simulink model "springScale_sith_weights"  (R2023a)
settings: Solver=VariableStepAuto  StartTime=0.0  StopTime=20.0  RelTol=1e-3
undefined symbols (not defined in the file or in its folder): c, k1, k2, m, x0
settings Model: Creator=kawat  LastModifiedBy=kawat

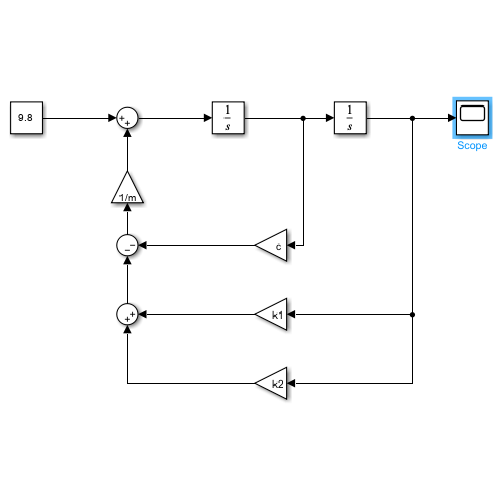
[thumbnail: Simulink's stored preview of the top-level diagram]
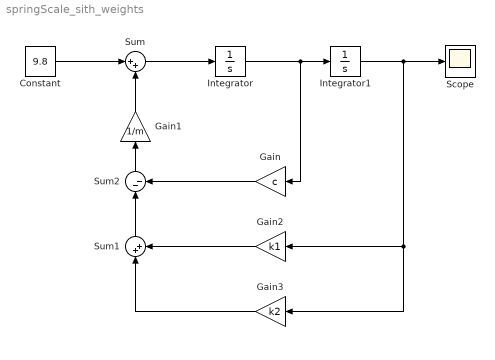
== system springScale_sith_weights ==
  Constant : Constant  Value=9.8  SampleTime=0.001
  Gain : Gain  Gain=c
  Gain1 : Gain  Gain=1/m
  Gain2 : Gain  Gain=k1
  Gain3 : Gain  Gain=k2
  Integrator : Integrator
  Integrator1 : Integrator  InitialCondition=x0
  Scope : Scope
  Sum : Sum  Inputs=|++
  Sum1 : Sum  Inputs=|++
  Sum2 : Sum  Inputs=|--
  wires:
  Constant/1 -> Sum/1
  Gain1/1 -> Sum/2
  Sum2/1 -> Gain1/1
  Sum1/1 -> Sum2/1
  Sum/1 -> Integrator/1
  Integrator/1 -> Gain/1, Integrator1/1
  Gain/1 -> Sum2/2
  Gain2/1 -> Sum1/2
  Gain3/1 -> Sum1/1
  Integrator1/1 -> Gain3/1, Gain2/1, Scope/1
